simulink model "discrete_starmac"  (Simulink 6.6)
settings: Solver=FixedStepDiscrete  StartTime=0.0  StopTime=10.0  FixedStep=plant_int_period  RelTol=1e-3
values from neighbouring files (symbols this model uses):
  A = pi*R^2    (= 0.0506707479097)    [constants.m]
  b = 0.1    [constants.m]
  g = [0 0 9.8]'    [constants.m]
  J = [Jxx 0 0 ... (first row only)    [constants.m]
  K_a1s = .009    (= 0.009)    [constants.m]
  K_beta = 0.23    [constants.m]
  K_torque = 0.47    [constants.m]
  M = 1.8263    [constants.m]
  motor_noise = noise_on*(9.8/4*.05)^2    [constants.m]
  plant_int_period = t_s / tau_motor    (= 0.00131578947368)    [constants.m]
  r1 = [dx 0 -dz]'    [constants.m]
  r2 = [0 dx -dz]'    [constants.m]
  r3 = [-dx 0 -dz]'    [constants.m]
  r4 = [0 -dx -dz]'    [constants.m]
  R_90 = [0 -1 0 ... (first row only)    [constants.m]
  rho = 1.2    [constants.m]
  T_nom = M*9.8/4    (= 4.474435)    [constants.m]
  tau_motor = 10    [constants.m]
  thrust_max = 9.8 * 1    (= 9.8)    [constants.m]
  thrust_min = 0    [constants.m]
  v_min = 1e-3    (= 0.001)    [constants.m]
libraries: simulink x13, xpcmeasurementcomputinglib x5, xpclib x3, aero_sim_lib x1
settings Model: Creator=jporter  LastModifiedBy=Administrator  BufferReuse=off  ProdHWDeviceType=Generic->32-bit x86 compatible
settings DataIOCC: LimitDataPoints=off  SaveOutput=off  SignalLogging=off  SaveTime=off
settings OptimizationCC: BlockReduction=off  OptimizeBlockIOStorage=off  BufferReuse=off  ExpressionFolding=off  LocalBlockOutputs=off
settings HardwareCC: ProdIntDivRoundTo=Zero  ProdEndianess=LittleEndian  ProdHWDeviceType=Generic->32-bit x86 compatible
settings RTWCC: SystemTargetFile=xpctarget.tlc  TemplateMakefile=xpc_default_tmf  Description=xPC Target  ProcessScript=xpctarget_make_rtw_hook
settings xpcTargetCC: TargetFcnLib=ansi_tfl_table_tmw.mat  GenFloatMathFcnCalls=ANSI_C  PortableWordSizes=off  xPCisDownloadable=off

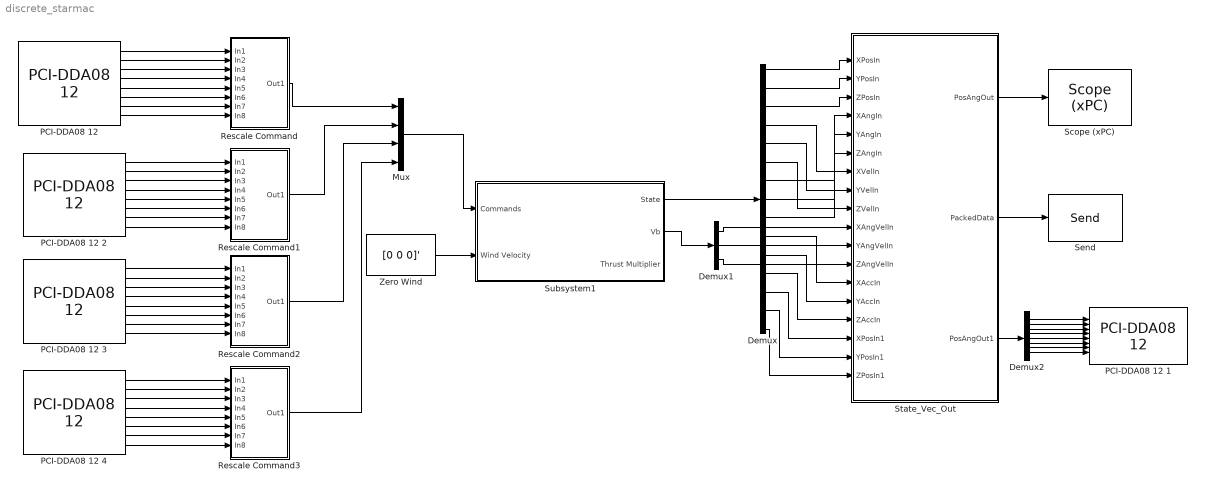
== system discrete_starmac ==
  Demux : Demux  Outputs=15
  Demux1 : Demux  Outputs=3
  Demux2 : Demux  Outputs=8
  Mux : Mux
  "PCI-DDA08 12 " : xpcmeasurementcomputinglib/Digital Input/PCI-DDA08 12   channel=[1 2 3 4 5 6 7 8]  port=A  chip=1  sampletime=plant_int_period  slot=-1
  PCI-DDA08 12 1 : xpcmeasurementcomputinglib/D//A/PCI-DDA08 12   channel=[1 2 3 4 5 6 7 8]  range=[-10 -10 -10 -10 -10 -10 -10 -10]  reset=[1]  initValue=[0]  sampletime=plant_int_period  pci_dev=-1
  PCI-DDA08 12 2 : xpcmeasurementcomputinglib/Digital Input/PCI-DDA08 12   channel=[1 2 3 4 5 6 7 8]  port=B  chip=1  sampletime=plant_int_period  slot=-1
  PCI-DDA08 12 3 : xpcmeasurementcomputinglib/Digital Input/PCI-DDA08 12   channel=[1 2 3 4 5 6 7 8]  port=A  chip=2  sampletime=plant_int_period  slot=-1
  PCI-DDA08 12 4 : xpcmeasurementcomputinglib/Digital Input/PCI-DDA08 12   channel=[1 2 3 4 5 6 7 8]  port=B  chip=2  sampletime=plant_int_period  slot=-1
  Rescale Command : Subsystem
  Rescale Command1 : Subsystem
  Rescale Command2 : Subsystem
  Rescale Command3 : Subsystem
  "Scope (xPC) " : xpclib/Misc./Scope (xPC)   SystemSampleTime=-1  scopeno=2  scopetype=Target  autostart=on  viewmode=Graphical redraw  formatstr='%15.6f'  grid=on  ylimits=[-12,12]  nosamples=250  noprepostsamples=0  interleave=1  triggermode=FreeRun  triggersignal=1  triggerlevel=0.0  triggerslope=Either  triggerscope=1  triggersample=0  filename=data.dat  mode=Lazy  writesize=512  autorestart=off
  Send : xpclib/UDP/Send  ipAddress=129.59.129.186  ipPort=9877  localPort=-1  sampletime=0.05
  State_Vec_Out : Subsystem
  Subsystem1 : Subsystem
  Zero Wind : Constant  Value=[0 0 0]'
  wires:
  Mux/1 -> Subsystem1/1(Commands)
  Zero Wind/1 -> Subsystem1/2(Wind Velocity)
  State_Vec_Out/1(PosAngOut) -> "Scope (xPC) "/1
  State_Vec_Out/2(PackedData) -> Send/1
  Subsystem1/1(State) -> Demux/1
  Demux/1 -> State_Vec_Out/1(XPosIn)
  Demux/2 -> State_Vec_Out/2(YPosIn)
  Demux/3 -> State_Vec_Out/3(ZPosIn)
  Demux/4 -> State_Vec_Out/7(XVelIn)
  Demux/5 -> State_Vec_Out/8(YVelIn)
  Demux/6 -> State_Vec_Out/9(ZVelIn)
  Demux/7 -> State_Vec_Out/4(XAngIn)
  Demux/8 -> State_Vec_Out/5(YAngIn)
  Demux/9 -> State_Vec_Out/6(ZAngIn)
  Demux/10 -> State_Vec_Out/13(XAccIn)
  Demux/11 -> State_Vec_Out/14(YAccIn)
  Demux/12 -> State_Vec_Out/15(ZAccIn)
  Demux/13 -> State_Vec_Out/16(XPosIn1)
  Demux/14 -> State_Vec_Out/17(YPosIn1)
  Demux/15 -> State_Vec_Out/18(ZPosIn1)
  Demux1/1 -> State_Vec_Out/10(XAngVelIn)
  Demux1/2 -> State_Vec_Out/11(YAngVelIn)
  Demux1/3 -> State_Vec_Out/12(ZAngVelIn)
  Subsystem1/2(Vb) -> Demux1/1
  Demux2/1 -> PCI-DDA08 12 1/1
  Demux2/2 -> PCI-DDA08 12 1/2
  Demux2/3 -> PCI-DDA08 12 1/3
  Demux2/4 -> PCI-DDA08 12 1/4
  Demux2/5 -> PCI-DDA08 12 1/5
  Demux2/6 -> PCI-DDA08 12 1/6
  Demux2/7 -> PCI-DDA08 12 1/7
  Demux2/8 -> PCI-DDA08 12 1/8
  State_Vec_Out/3(PosAngOut1) -> Demux2/1
  "PCI-DDA08 12 "/1 -> Rescale Command/1(In1)
  "PCI-DDA08 12 "/2 -> Rescale Command/2(In2)
  "PCI-DDA08 12 "/3 -> Rescale Command/3(In3)
  "PCI-DDA08 12 "/4 -> Rescale Command/4(In4)
  "PCI-DDA08 12 "/5 -> Rescale Command/5(In5)
  "PCI-DDA08 12 "/6 -> Rescale Command/6(In6)
  "PCI-DDA08 12 "/7 -> Rescale Command/7(In7)
  "PCI-DDA08 12 "/8 -> Rescale Command/8(In8)
  Rescale Command/1(Out1) -> Mux/1
  PCI-DDA08 12 2/1 -> Rescale Command1/1(In1)
  PCI-DDA08 12 2/2 -> Rescale Command1/2(In2)
  PCI-DDA08 12 2/3 -> Rescale Command1/3(In3)
  PCI-DDA08 12 2/4 -> Rescale Command1/4(In4)
  PCI-DDA08 12 2/5 -> Rescale Command1/5(In5)
  PCI-DDA08 12 2/6 -> Rescale Command1/6(In6)
  PCI-DDA08 12 2/7 -> Rescale Command1/7(In7)
  PCI-DDA08 12 2/8 -> Rescale Command1/8(In8)
  PCI-DDA08 12 3/1 -> Rescale Command2/1(In1)
  PCI-DDA08 12 3/2 -> Rescale Command2/2(In2)
  PCI-DDA08 12 3/3 -> Rescale Command2/3(In3)
  PCI-DDA08 12 3/4 -> Rescale Command2/4(In4)
  PCI-DDA08 12 3/5 -> Rescale Command2/5(In5)
  PCI-DDA08 12 3/6 -> Rescale Command2/6(In6)
  PCI-DDA08 12 3/7 -> Rescale Command2/7(In7)
  PCI-DDA08 12 3/8 -> Rescale Command2/8(In8)
  PCI-DDA08 12 4/1 -> Rescale Command3/1(In1)
  PCI-DDA08 12 4/2 -> Rescale Command3/2(In2)
  PCI-DDA08 12 4/3 -> Rescale Command3/3(In3)
  PCI-DDA08 12 4/4 -> Rescale Command3/4(In4)
  PCI-DDA08 12 4/5 -> Rescale Command3/5(In5)
  PCI-DDA08 12 4/6 -> Rescale Command3/6(In6)
  PCI-DDA08 12 4/7 -> Rescale Command3/7(In7)
  PCI-DDA08 12 4/8 -> Rescale Command3/8(In8)
  Rescale Command1/1(Out1) -> Mux/2
  Rescale Command2/1(Out1) -> Mux/3
  Rescale Command3/1(Out1) -> Mux/4

== system discrete_starmac/Rescale Command ==
  In1 : Inport  OutDataType=fixdt(1,16,0)  OutScaling=[]
  In2 : Inport  Port=2  OutDataType=fixdt(1,16,0)  OutScaling=[]
  In3 : Inport  Port=3  OutDataType=fixdt(1,16,0)  OutScaling=[]
  In4 : Inport  Port=4  OutDataType=fixdt(1,16,0)  OutScaling=[]
  In5 : Inport  Port=5  OutDataType=fixdt(1,16,0)  OutScaling=[]
  In6 : Inport  Port=6  OutDataType=fixdt(1,16,0)  OutScaling=[]
  In7 : Inport  Port=7  OutDataType=fixdt(1,16,0)  OutScaling=[]
  In8 : Inport  Port=8  OutDataType=fixdt(1,16,0)  OutScaling=[]
  Constant : Constant  Value=(2*ones(1,8)).^[7:-1:0]
  Dot Product : simulink/Math Operations/Dot Product  InputSameDT=on  OutDataType=sfix(16)  OutScaling=2^-10  DoSatur=off
  Mux1 : Mux  Inputs=8
  Rescale : Gain
  Out1 : Outport  OutDataType=fixdt(1,16,0)  OutScaling=[]
  wires:
  Mux1/1 -> Dot Product/2
  Constant/1 -> Dot Product/1
  Dot Product/1 -> Rescale/1
  In1/1 -> Mux1/1
  In2/1 -> Mux1/2
  In3/1 -> Mux1/3
  In4/1 -> Mux1/4
  In5/1 -> Mux1/5
  In6/1 -> Mux1/6
  In7/1 -> Mux1/7
  In8/1 -> Mux1/8
  Rescale/1 -> Out1/1

== system discrete_starmac/Rescale Command1 ==
  In1 : Inport  OutDataType=fixdt(1,16,0)  OutScaling=[]
  In2 : Inport  Port=2  OutDataType=fixdt(1,16,0)  OutScaling=[]
  In3 : Inport  Port=3  OutDataType=fixdt(1,16,0)  OutScaling=[]
  In4 : Inport  Port=4  OutDataType=fixdt(1,16,0)  OutScaling=[]
  In5 : Inport  Port=5  OutDataType=fixdt(1,16,0)  OutScaling=[]
  In6 : Inport  Port=6  OutDataType=fixdt(1,16,0)  OutScaling=[]
  In7 : Inport  Port=7  OutDataType=fixdt(1,16,0)  OutScaling=[]
  In8 : Inport  Port=8  OutDataType=fixdt(1,16,0)  OutScaling=[]
  Constant : Constant  Value=(2*ones(1,8)).^[7:-1:0]
  Dot Product : simulink/Math Operations/Dot Product  InputSameDT=on  OutDataType=sfix(16)  OutScaling=2^-10  DoSatur=off
  Mux1 : Mux  Inputs=8
  Rescale : Gain
  Out1 : Outport  OutDataType=fixdt(1,16,0)  OutScaling=[]
  wires:
  Mux1/1 -> Dot Product/2
  Constant/1 -> Dot Product/1
  Dot Product/1 -> Rescale/1
  In1/1 -> Mux1/1
  In2/1 -> Mux1/2
  In3/1 -> Mux1/3
  In4/1 -> Mux1/4
  In5/1 -> Mux1/5
  In6/1 -> Mux1/6
  In7/1 -> Mux1/7
  In8/1 -> Mux1/8
  Rescale/1 -> Out1/1

== system discrete_starmac/Rescale Command2 ==
  In1 : Inport  OutDataType=fixdt(1,16,0)  OutScaling=[]
  In2 : Inport  Port=2  OutDataType=fixdt(1,16,0)  OutScaling=[]
  In3 : Inport  Port=3  OutDataType=fixdt(1,16,0)  OutScaling=[]
  In4 : Inport  Port=4  OutDataType=fixdt(1,16,0)  OutScaling=[]
  In5 : Inport  Port=5  OutDataType=fixdt(1,16,0)  OutScaling=[]
  In6 : Inport  Port=6  OutDataType=fixdt(1,16,0)  OutScaling=[]
  In7 : Inport  Port=7  OutDataType=fixdt(1,16,0)  OutScaling=[]
  In8 : Inport  Port=8  OutDataType=fixdt(1,16,0)  OutScaling=[]
  Constant : Constant  Value=(2*ones(1,8)).^[7:-1:0]
  Dot Product : simulink/Math Operations/Dot Product  InputSameDT=on  OutDataType=sfix(16)  OutScaling=2^-10  DoSatur=off
  Mux1 : Mux  Inputs=8
  Rescale : Gain
  Out1 : Outport  OutDataType=fixdt(1,16,0)  OutScaling=[]
  wires:
  Mux1/1 -> Dot Product/2
  Constant/1 -> Dot Product/1
  Dot Product/1 -> Rescale/1
  In1/1 -> Mux1/1
  In2/1 -> Mux1/2
  In3/1 -> Mux1/3
  In4/1 -> Mux1/4
  In5/1 -> Mux1/5
  In6/1 -> Mux1/6
  In7/1 -> Mux1/7
  In8/1 -> Mux1/8
  Rescale/1 -> Out1/1

== system discrete_starmac/Rescale Command3 ==
  In1 : Inport  OutDataType=fixdt(1,16,0)  OutScaling=[]
  In2 : Inport  Port=2  OutDataType=fixdt(1,16,0)  OutScaling=[]
  In3 : Inport  Port=3  OutDataType=fixdt(1,16,0)  OutScaling=[]
  In4 : Inport  Port=4  OutDataType=fixdt(1,16,0)  OutScaling=[]
  In5 : Inport  Port=5  OutDataType=fixdt(1,16,0)  OutScaling=[]
  In6 : Inport  Port=6  OutDataType=fixdt(1,16,0)  OutScaling=[]
  In7 : Inport  Port=7  OutDataType=fixdt(1,16,0)  OutScaling=[]
  In8 : Inport  Port=8  OutDataType=fixdt(1,16,0)  OutScaling=[]
  Constant : Constant  Value=(2*ones(1,8)).^[7:-1:0]
  Dot Product : simulink/Math Operations/Dot Product  InputSameDT=on  OutDataType=sfix(16)  OutScaling=2^-10  DoSatur=off
  Mux1 : Mux  Inputs=8
  Rescale : Gain
  Out1 : Outport  OutDataType=fixdt(1,16,0)  OutScaling=[]
  wires:
  Mux1/1 -> Dot Product/2
  Constant/1 -> Dot Product/1
  Dot Product/1 -> Rescale/1
  In1/1 -> Mux1/1
  In2/1 -> Mux1/2
  In3/1 -> Mux1/3
  In4/1 -> Mux1/4
  In5/1 -> Mux1/5
  In6/1 -> Mux1/6
  In7/1 -> Mux1/7
  In8/1 -> Mux1/8
  Rescale/1 -> Out1/1

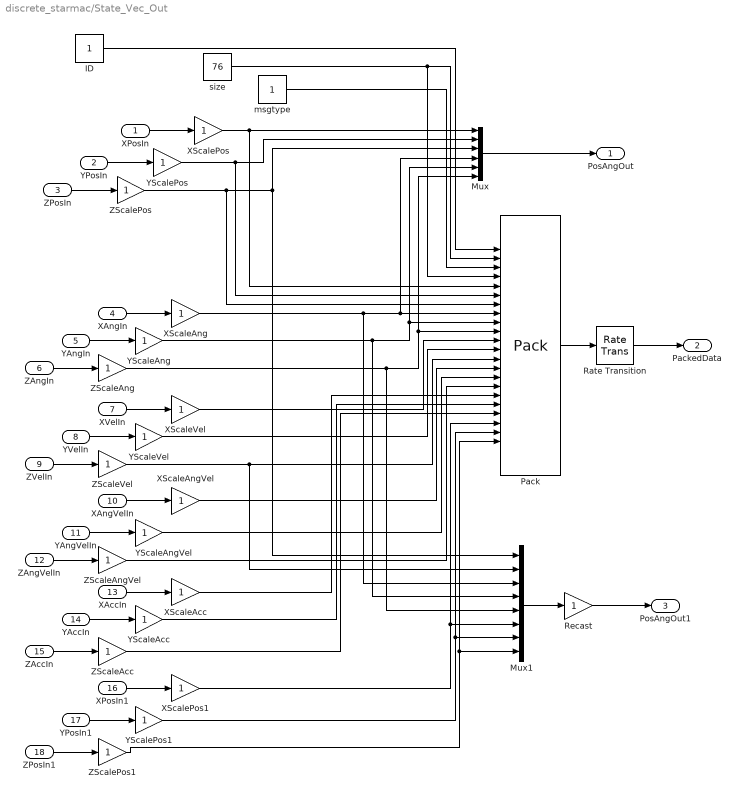
== system discrete_starmac/State_Vec_Out ==
  XPosIn : Inport
  YPosIn : Inport  Port=2
  ZPosIn : Inport  Port=3
  XAngIn : Inport  Port=4
  YAngIn : Inport  Port=5
  ZAngIn : Inport  Port=6
  XVelIn : Inport  Port=7
  YVelIn : Inport  Port=8
  ZVelIn : Inport  Port=9
  XAngVelIn : Inport  Port=10
  YAngVelIn : Inport  Port=11
  ZAngVelIn : Inport  Port=12
  XAccIn : Inport  Port=13
  YAccIn : Inport  Port=14
  ZAccIn : Inport  Port=15
  XPosIn1 : Inport  Port=16
  YPosIn1 : Inport  Port=17
  ZPosIn1 : Inport  Port=18
  ID : Constant
  Mux : Mux  Inputs=6
  Mux1 : Mux  Inputs=8
  Pack : xpclib/UDP/Pack  datatypes={'uint32','uint32','uint32','uint32','single','single','single','single','single','single','single','single','single','single','single','single','single','single','single','single','single','single'}  byteAlign=4
  Rate Transition : RateTransition
  Recast : Gain
  XScaleAcc : Gain
  XScaleAng : Gain
  XScaleAngVel : Gain
  XScalePos : Gain
  XScalePos1 : Gain
  XScaleVel : Gain
  YScaleAcc : Gain
  YScaleAng : Gain
  YScaleAngVel : Gain
  YScalePos : Gain
  YScalePos1 : Gain
  YScaleVel : Gain
  ZScaleAcc : Gain
  ZScaleAng : Gain
  ZScaleAngVel : Gain
  ZScalePos : Gain
  ZScalePos1 : Gain
  ZScaleVel : Gain
  msgtype : Constant
  size : Constant  Value=76
  PosAngOut : Outport
  PackedData : Outport  Port=2
  PosAngOut1 : Outport  Port=3
  wires:
  Pack/1 -> Rate Transition/1
  XScaleAng/1 -> Mux/4, Pack/8, Mux1/3
  YScaleAng/1 -> Mux/5, Pack/9, Mux1/4
  ZScaleAng/1 -> Mux/6, Pack/10, Mux1/5
  ID/1 -> Pack/1
  size/1 -> Pack/2, Pack/4
  msgtype/1 -> Pack/3
  XScaleVel/1 -> Pack/11
  YScaleVel/1 -> Pack/12
  ZScaleVel/1 -> Pack/13, Mux1/2
  XScaleAngVel/1 -> Pack/14
  YScaleAngVel/1 -> Pack/15
  ZScaleAngVel/1 -> Pack/16
  XScaleAcc/1 -> Pack/17
  YScaleAcc/1 -> Pack/18
  ZScaleAcc/1 -> Pack/19
  XScalePos1/1 -> Pack/20, Mux1/6
  YScalePos1/1 -> Pack/21, Mux1/7
  ZScalePos1/1 -> Pack/22, Mux1/8
  Mux/1 -> PosAngOut/1
  XPosIn/1 -> XScalePos/1
  YPosIn/1 -> YScalePos/1
  ZPosIn/1 -> ZScalePos/1
  XScalePos/1 -> Mux/1, Pack/5
  YScalePos/1 -> Mux/2, Pack/6
  ZScalePos/1 -> Pack/7, Mux/3, Mux1/1
  XAngIn/1 -> XScaleAng/1
  YAngIn/1 -> YScaleAng/1
  ZAngIn/1 -> ZScaleAng/1
  XVelIn/1 -> XScaleVel/1
  YVelIn/1 -> YScaleVel/1
  ZVelIn/1 -> ZScaleVel/1
  XAngVelIn/1 -> XScaleAngVel/1
  YAngVelIn/1 -> YScaleAngVel/1
  ZAngVelIn/1 -> ZScaleAngVel/1
  XAccIn/1 -> XScaleAcc/1
  YAccIn/1 -> YScaleAcc/1
  ZAccIn/1 -> ZScaleAcc/1
  XPosIn1/1 -> XScalePos1/1
  YPosIn1/1 -> YScalePos1/1
  ZPosIn1/1 -> ZScalePos1/1
  Rate Transition/1 -> PackedData/1
  Mux1/1 -> Recast/1
  Recast/1 -> PosAngOut1/1

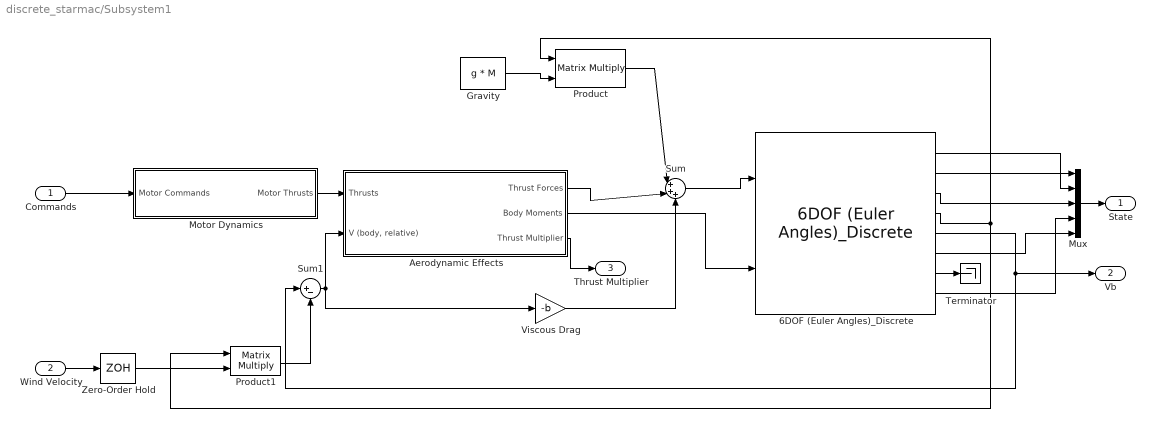
== system discrete_starmac/Subsystem1 ==
  Commands : Inport
  Wind Velocity : Inport  Port=2
  6DOF (Euler Angles)_Discrete : aero_sim_lib/6DOF (Euler Angles)_Discrete  SystemSampleTime=-1  XYZe_0=X0  Vb_0=Vb0  euler_0=T0  omega_0=W0  M=M  I=J  T_int=plant_int_period
  Aerodynamic Effects : Subsystem
  Gravity : Constant  Value=g * M
  Motor Dynamics : Subsystem
  Mux : Mux  Inputs=5
  Product : Product  Multiplication=Matrix(*)  RndMeth=Zero
  Product1 : Product  Multiplication=Matrix(*)  RndMeth=Zero
  Sum : Sum  Inputs=|+++
  Sum1 : Sum  Inputs=|+-
  Terminator : Terminator
  Viscous Drag : Gain  Gain=-b
  Zero-Order Hold : ZeroOrderHold  SampleTime=plant_int_period
  State : Outport
  Vb : Outport  Port=2
  Thrust Multiplier : Outport  Port=3
  wires:
  Motor Dynamics/1(Motor Thrusts) -> Aerodynamic Effects/1(Thrusts)
  Product/1 -> Sum/1
  Sum/1 -> 6DOF (Euler Angles)_Discrete/1
  6DOF (Euler Angles)_Discrete/4 -> Product/1, Product1/1
  Gravity/1 -> Product/2
  Sum1/1 -> Aerodynamic Effects/2("V (body, relative)"), Viscous Drag/1
  Product1/1 -> Sum1/2
  6DOF (Euler Angles)_Discrete/5 -> Sum1/1, Vb/1
  Viscous Drag/1 -> Sum/3
  6DOF (Euler Angles)_Discrete/2 -> Mux/1
  6DOF (Euler Angles)_Discrete/1 -> Mux/2
  6DOF (Euler Angles)_Discrete/3 -> Mux/3
  Aerodynamic Effects/2(Body Moments) -> 6DOF (Euler Angles)_Discrete/2
  Aerodynamic Effects/1(Thrust Forces) -> Sum/2
  Mux/1 -> State/1
  Commands/1 -> Motor Dynamics/1(Motor Commands)
  Wind Velocity/1 -> Zero-Order Hold/1
  Aerodynamic Effects/3(Thrust Multiplier) -> Thrust Multiplier/1
  6DOF (Euler Angles)_Discrete/8 -> Mux/4
  Zero-Order Hold/1 -> Product1/2
  6DOF (Euler Angles)_Discrete/7 -> Terminator/1
  6DOF (Euler Angles)_Discrete/6 -> Mux/5

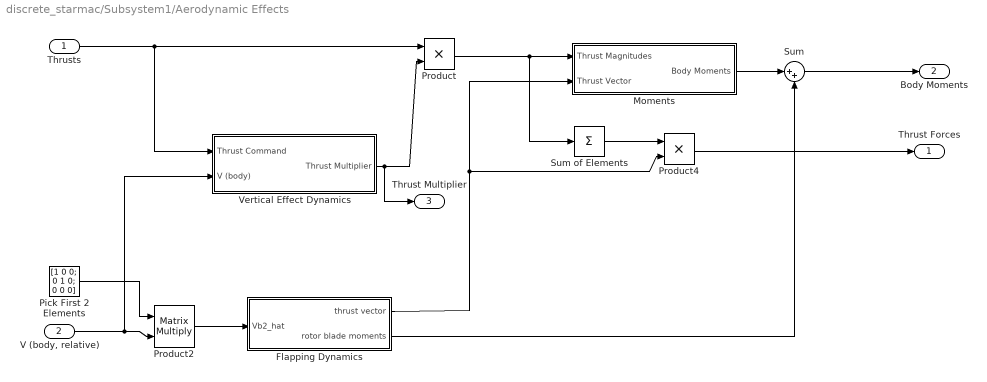
== system discrete_starmac/Subsystem1/Aerodynamic Effects ==
  Thrusts : Inport
  "V (body, relative)" : Inport  Port=2
  Flapping Dynamics : Subsystem
  Moments : Subsystem
  Pick First 2 Elements : Constant  Value=[1 0 0; 0 1 0; 0 0 0]
  Product : Product  RndMeth=Zero
  Product2 : Product  Multiplication=Matrix(*)  RndMeth=Zero
  Product4 : Product  RndMeth=Zero
  Sum : Sum  Inputs=|++
  Sum of Elements : Sum  Inputs=+  OutScaling=2^-10
  Vertical Effect Dynamics : Subsystem
  Thrust Forces : Outport
  Body Moments : Outport  Port=2
  Thrust Multiplier : Outport  Port=3
  wires:
  Thrusts/1 -> Product/1, Vertical Effect Dynamics/1(Thrust Command)
  Vertical Effect Dynamics/1(Thrust Multiplier) -> Product/2, Thrust Multiplier/1
  Product/1 -> Sum of Elements/1, Moments/1(Thrust Magnitudes)
  Pick First 2 Elements/1 -> Product2/1
  "V (body, relative)"/1 -> Product2/2, Vertical Effect Dynamics/2(V (body))
  Product2/1 -> Flapping Dynamics/1(Vb2_hat)
  Sum of Elements/1 -> Product4/1
  Product4/1 -> Thrust Forces/1
  Flapping Dynamics/1(thrust vector) -> Moments/2(Thrust Vector), Product4/2
  Moments/1(Body Moments) -> Sum/1
  Sum/1 -> Body Moments/1
  Flapping Dynamics/2(rotor blade moments) -> Sum/2

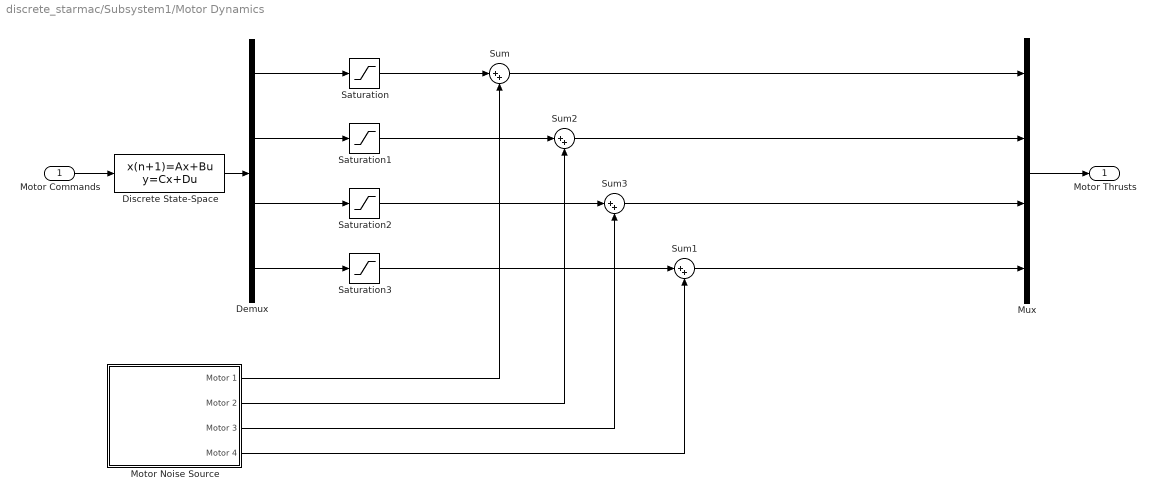
== system discrete_starmac/Subsystem1/Motor Dynamics ==
  Motor Commands : Inport
  Demux : Demux
  Discrete State-Space : DiscreteStateSpace  A=expm( -(tau_motor*plant_int_period) * eye(4) )  B=inv(expm( tau_motor * plant_int_period* eye(4))) * (expm((tau_motor*plant_int_period) * eye(4)) - eye(4))  C=eye(4)  D=zeros(4)  X0=T_nom * ones(4,1)  SampleTime=plant_int_period
  Motor Noise Source : Subsystem
  Mux : Mux
  Saturation{,1..3} (4 alike) : Saturate  UpperLimit=thrust_max  LowerLimit=thrust_min
  Sum{,1..3} (4 alike) : Sum  Inputs=|++
  Motor Thrusts : Outport
  wires:
  Demux/1 -> Saturation/1
  Demux/3 -> Saturation2/1
  Mux/1 -> Motor Thrusts/1
  Saturation/1 -> Sum/1
  Sum/1 -> Mux/1
  Saturation1/1 -> Sum2/1
  Sum2/1 -> Mux/2
  Saturation2/1 -> Sum3/1
  Sum3/1 -> Mux/3
  Saturation3/1 -> Sum1/1
  Sum1/1 -> Mux/4
  Motor Noise Source/1(Motor 1) -> Sum/2
  Motor Noise Source/2(Motor 2) -> Sum2/2
  Motor Noise Source/3(Motor 3) -> Sum3/2
  Motor Noise Source/4(Motor 4) -> Sum1/2
  Motor Commands/1 -> Discrete State-Space/1
  Discrete State-Space/1 -> Demux/1
  Demux/2 -> Saturation1/1
  Demux/4 -> Saturation3/1

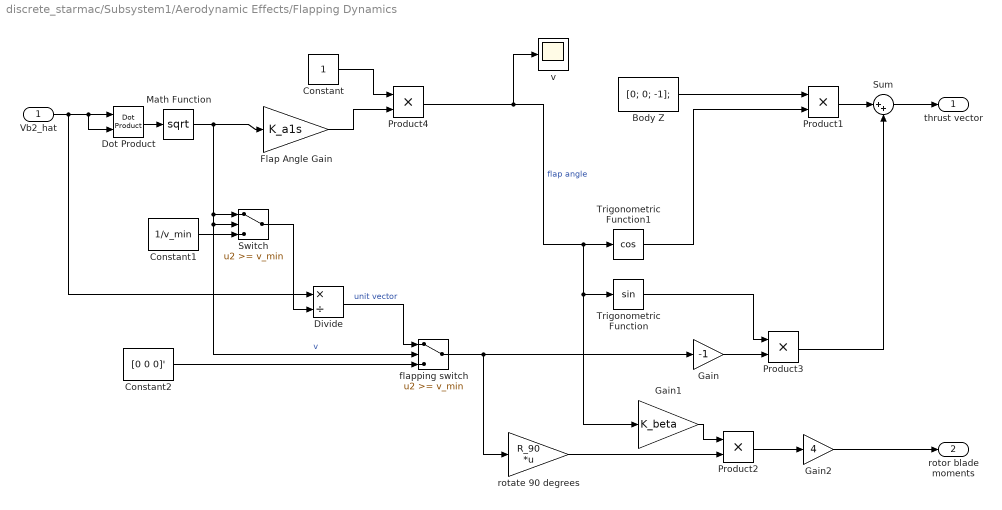
== system discrete_starmac/Subsystem1/Aerodynamic Effects/Flapping Dynamics ==
  Vb2_hat : Inport
  "Body Z " : Constant  Value=[0; 0; -1];
  Constant : Constant
  Constant1 : Constant  Value=1/v_min
  Constant2 : Constant  Value=[0 0 0]'
  Divide : Product  Inputs=*/  OutScaling=2^-10
  Dot Product : simulink/Math Operations/Dot Product  InputSameDT=on  OutDataType=sfix(16)  OutScaling=2^-10  DoSatur=off
  Flap Angle Gain : Gain  Gain=K_a1s
  Gain : Gain  Gain=-1
  Gain1 : Gain  Gain=K_beta
  Gain2 : Gain  Gain=4
  Math Function : Math  Operator=sqrt  SaturateOnIntegerOverflow=on
  Product{1..4} (4 alike) : Product  RndMeth=Zero
  Sum : Sum  Inputs=|++
  Switch : Switch  Threshold=v_min
  Trigonometric Function : Trigonometry
  Trigonometric Function1 : Trigonometry  Operator=cos
  flapping switch : Switch  Threshold=v_min
  rotate 90 degrees : Gain  Gain=R_90  Multiplication=Matrix(K*u)
  v : Scope
      settings: SaveName=ScopeData6
  thrust vector : Outport
  rotor blade moments : Outport  Port=2
  wires:
  Product4/1 -> Trigonometric Function1/1, Trigonometric Function/1, Gain1/1, v/1  "flap angle"
  Vb2_hat/1 -> Dot Product/1, Dot Product/2, Divide/1
  Dot Product/1 -> Math Function/1
  Math Function/1 -> Switch/1, Switch/2, flapping switch/2, Flap Angle Gain/1  "v"
  Trigonometric Function1/1 -> Product1/2
  Trigonometric Function/1 -> Product3/1
  Product3/1 -> Sum/2
  Gain/1 -> Product3/2
  Product1/1 -> Sum/1
  "Body Z "/1 -> Product1/1
  Sum/1 -> thrust vector/1
  Gain2/1 -> rotor blade moments/1
  Switch/1 -> Divide/2
  Constant1/1 -> Switch/3
  Divide/1 -> flapping switch/1  "unit vector"
  flapping switch/1 -> Gain/1, rotate 90 degrees/1
  Constant2/1 -> flapping switch/3
  Product2/1 -> Gain2/1
  rotate 90 degrees/1 -> Product2/2
  Gain1/1 -> Product2/1
  Flap Angle Gain/1 -> Product4/2
  Constant/1 -> Product4/1

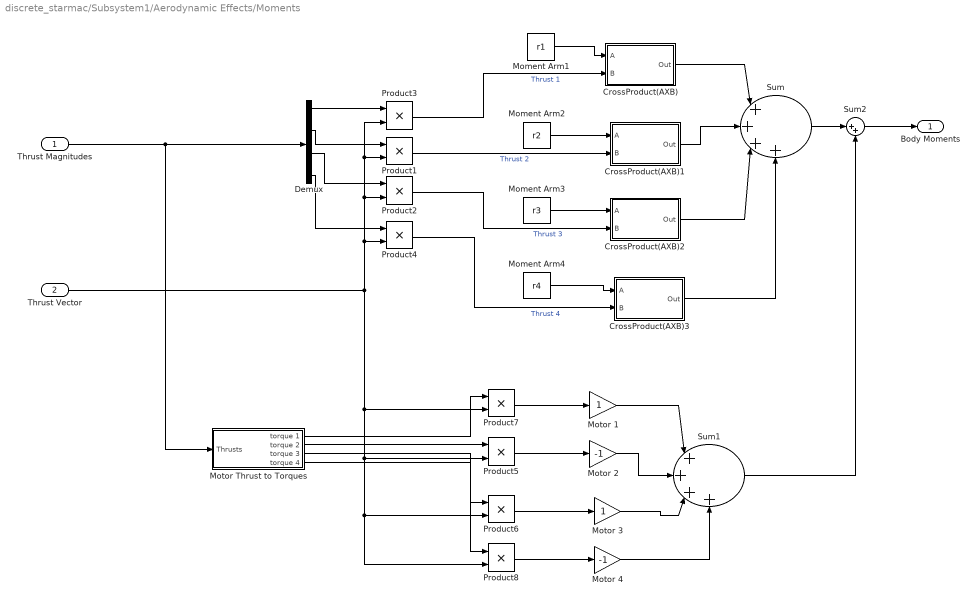
== system discrete_starmac/Subsystem1/Aerodynamic Effects/Moments ==
  Thrust Magnitudes : Inport
  Thrust Vector : Inport  Port=2
  CrossProduct(AXB) : Subsystem
  CrossProduct(AXB)1 : Subsystem
  CrossProduct(AXB)2 : Subsystem
  CrossProduct(AXB)3 : Subsystem
  Demux : Demux
  Moment Arm1 : Constant  Value=r1
  Moment Arm2 : Constant  Value=r2
  Moment Arm3 : Constant  Value=r3
  Moment Arm4 : Constant  Value=r4
  Motor 1 : Gain
  Motor 2 : Gain  Gain=-1
  Motor 3 : Gain
  Motor 4 : Gain  Gain=-1
  Motor Thrust to Torques : Subsystem
  Product{1..8} (8 alike) : Product  RndMeth=Zero
  Sum : Sum  Inputs=|++++
  Sum1 : Sum  Inputs=|++++
  Sum2 : Sum  Inputs=|++
  Body Moments : Outport
  wires:
  Thrust Magnitudes/1 -> Demux/1, Motor Thrust to Torques/1(Thrusts)
  Demux/1 -> Product3/1
  Demux/2 -> Product1/1
  Demux/3 -> Product2/1
  Demux/4 -> Product4/1
  Thrust Vector/1 -> Product3/2, Product1/2, Product2/2, Product4/2, Product7/2, Product5/2, Product6/2, Product8/2
  Moment Arm1/1 -> CrossProduct(AXB)/1(A)
  Product3/1 -> CrossProduct(AXB)/2(B)  "Thrust 1"
  Moment Arm2/1 -> CrossProduct(AXB)1/1(A)
  Product1/1 -> CrossProduct(AXB)1/2(B)  "Thrust 2"
  Moment Arm3/1 -> CrossProduct(AXB)2/1(A)
  Product2/1 -> CrossProduct(AXB)2/2(B)  "Thrust 3"
  Moment Arm4/1 -> CrossProduct(AXB)3/1(A)
  Product4/1 -> CrossProduct(AXB)3/2(B)  "Thrust 4"
  CrossProduct(AXB)/1(Out) -> Sum/1
  CrossProduct(AXB)2/1(Out) -> Sum/3
  CrossProduct(AXB)3/1(Out) -> Sum/4
  Motor 1/1 -> Sum1/1
  Motor 2/1 -> Sum1/2
  Motor 3/1 -> Sum1/3
  Motor 4/1 -> Sum1/4
  Sum/1 -> Sum2/1
  Sum1/1 -> Sum2/2
  Sum2/1 -> Body Moments/1
  Product7/1 -> Motor 1/1
  Product5/1 -> Motor 2/1
  Product6/1 -> Motor 3/1
  Product8/1 -> Motor 4/1
  Motor Thrust to Torques/1(torque 1) -> Product7/1
  Motor Thrust to Torques/2(torque 2) -> Product5/1
  Motor Thrust to Torques/3(torque 3) -> Product6/1
  Motor Thrust to Torques/4(torque 4) -> Product8/1
  CrossProduct(AXB)1/1(Out) -> Sum/2

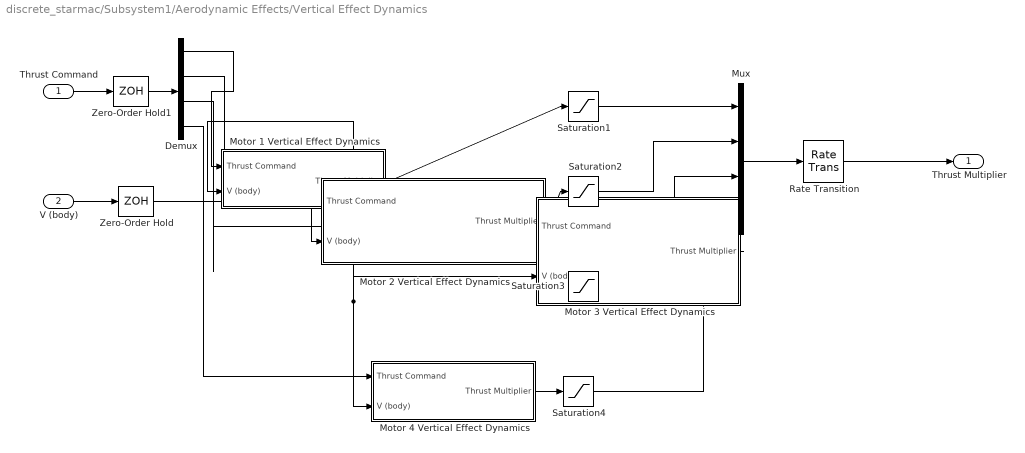
== system discrete_starmac/Subsystem1/Aerodynamic Effects/Vertical Effect Dynamics ==
  Thrust Command : Inport
  V (body) : Inport  Port=2
  Demux : Demux
  Motor 1 Vertical Effect Dynamics : Subsystem
  Motor 2 Vertical Effect Dynamics : Subsystem
  Motor 3 Vertical Effect Dynamics : Subsystem
  Motor 4 Vertical Effect Dynamics : Subsystem
  Mux : Mux
  Rate Transition : RateTransition
  Saturation{1..4} (4 alike) : Saturate  UpperLimit=2  LowerLimit=0.5
  Zero-Order Hold : ZeroOrderHold  SampleTime=plant_int_period*10
  Zero-Order Hold1 : ZeroOrderHold  SampleTime=plant_int_period*10
  Thrust Multiplier : Outport
  wires:
  Thrust Command/1 -> Zero-Order Hold1/1
  Mux/1 -> Rate Transition/1
  Demux/1 -> Motor 1 Vertical Effect Dynamics/1(Thrust Command)
  Demux/2 -> Motor 2 Vertical Effect Dynamics/1(Thrust Command)
  Demux/3 -> Motor 3 Vertical Effect Dynamics/1(Thrust Command)
  Demux/4 -> Motor 4 Vertical Effect Dynamics/1(Thrust Command)
  Motor 1 Vertical Effect Dynamics/1(Thrust Multiplier) -> Saturation1/1
  Motor 2 Vertical Effect Dynamics/1(Thrust Multiplier) -> Saturation2/1
  Motor 3 Vertical Effect Dynamics/1(Thrust Multiplier) -> Saturation3/1
  Motor 4 Vertical Effect Dynamics/1(Thrust Multiplier) -> Saturation4/1
  Saturation1/1 -> Mux/1
  Saturation2/1 -> Mux/2
  Saturation3/1 -> Mux/3
  Saturation4/1 -> Mux/4
  V (body)/1 -> Zero-Order Hold/1
  Zero-Order Hold/1 -> Motor 1 Vertical Effect Dynamics/2(V (body)), Motor 2 Vertical Effect Dynamics/2(V (body)), Motor 3 Vertical Effect Dynamics/2(V (body)), Motor 4 Vertical Effect Dynamics/2(V (body))
  Zero-Order Hold1/1 -> Demux/1
  Rate Transition/1 -> Thrust Multiplier/1

== system discrete_starmac/Subsystem1/Motor Dynamics/Motor Noise Source ==
  Motor Noise : RandomNumber  Variance=motor_noise  SampleTime=plant_int_period
  Motor Noise1 : RandomNumber  Variance=motor_noise  Seed=1  SampleTime=plant_int_period
  Motor Noise2 : RandomNumber  Variance=motor_noise  Seed=2  SampleTime=plant_int_period
  Motor Noise3 : RandomNumber  Variance=motor_noise  Seed=3  SampleTime=plant_int_period
  Motor 1 : Outport
  Motor 2 : Outport  Port=2
  Motor 3 : Outport  Port=3
  Motor 4 : Outport  Port=4
  wires:
  Motor Noise/1 -> Motor 1/1
  Motor Noise1/1 -> Motor 2/1
  Motor Noise2/1 -> Motor 3/1
  Motor Noise3/1 -> Motor 4/1

== system discrete_starmac/Subsystem1/Aerodynamic Effects/Moments/CrossProduct(AXB) ==
  A : Inport
  B : Inport  Port=2
  Fcn : Fcn  Expr=u[2]*u[6]-u[3]*u[5]
  Fcn1 : Fcn  Expr=u[3]*u[4]-u[1]*u[6]
  Fcn2 : Fcn  Expr=u[1]*u[5]-u[2]*u[4]
  Mux : Mux  Inputs=2
  Mux1 : Mux  Inputs=3
  Out : Outport
  wires:
  A/1 -> Mux/1
  B/1 -> Mux/2
  Mux/1 -> Fcn/1, Fcn1/1, Fcn2/1
  Fcn/1 -> Mux1/1
  Fcn1/1 -> Mux1/2
  Fcn2/1 -> Mux1/3
  Mux1/1 -> Out/1

== system discrete_starmac/Subsystem1/Aerodynamic Effects/Moments/CrossProduct(AXB)1 ==
  A : Inport
  B : Inport  Port=2
  Fcn : Fcn  Expr=u[2]*u[6]-u[3]*u[5]
  Fcn1 : Fcn  Expr=u[3]*u[4]-u[1]*u[6]
  Fcn2 : Fcn  Expr=u[1]*u[5]-u[2]*u[4]
  Mux : Mux  Inputs=2
  Mux1 : Mux  Inputs=3
  Out : Outport
  wires:
  Mux1/1 -> Out/1
  Fcn2/1 -> Mux1/3
  Fcn1/1 -> Mux1/2
  Fcn/1 -> Mux1/1
  Mux/1 -> Fcn2/1, Fcn1/1, Fcn/1
  B/1 -> Mux/2
  A/1 -> Mux/1

== system discrete_starmac/Subsystem1/Aerodynamic Effects/Moments/CrossProduct(AXB)2 ==
  A : Inport
  B : Inport  Port=2
  Fcn : Fcn  Expr=u[2]*u[6]-u[3]*u[5]
  Fcn1 : Fcn  Expr=u[3]*u[4]-u[1]*u[6]
  Fcn2 : Fcn  Expr=u[1]*u[5]-u[2]*u[4]
  Mux : Mux  Inputs=2
  Mux1 : Mux  Inputs=3
  Out : Outport
  wires:
  A/1 -> Mux/1
  B/1 -> Mux/2
  Mux/1 -> Fcn/1, Fcn1/1, Fcn2/1
  Fcn/1 -> Mux1/1
  Fcn1/1 -> Mux1/2
  Fcn2/1 -> Mux1/3
  Mux1/1 -> Out/1

== system discrete_starmac/Subsystem1/Aerodynamic Effects/Moments/CrossProduct(AXB)3 ==
  A : Inport
  B : Inport  Port=2
  Fcn : Fcn  Expr=u[2]*u[6]-u[3]*u[5]
  Fcn1 : Fcn  Expr=u[3]*u[4]-u[1]*u[6]
  Fcn2 : Fcn  Expr=u[1]*u[5]-u[2]*u[4]
  Mux : Mux  Inputs=2
  Mux1 : Mux  Inputs=3
  Out : Outport
  wires:
  Mux1/1 -> Out/1
  Fcn2/1 -> Mux1/3
  Fcn1/1 -> Mux1/2
  Fcn/1 -> Mux1/1
  Mux/1 -> Fcn2/1, Fcn1/1, Fcn/1
  B/1 -> Mux/2
  A/1 -> Mux/1

== system discrete_starmac/Subsystem1/Aerodynamic Effects/Moments/Motor Thrust to Torques ==
  Thrusts : Inport
  Demux : Demux
  Gain1 : Gain  Gain=K_torque
  torque 1 : Outport
  torque 2 : Outport  Port=2
  torque 3 : Outport  Port=3
  torque 4 : Outport  Port=4
  wires:
  Thrusts/1 -> Gain1/1
  Gain1/1 -> Demux/1
  Demux/1 -> torque 1/1
  Demux/2 -> torque 2/1
  Demux/3 -> torque 3/1
  Demux/4 -> torque 4/1

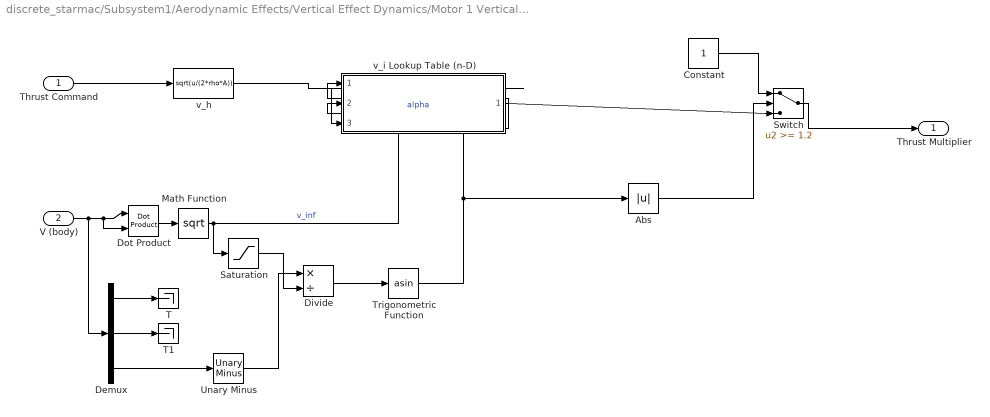
== system discrete_starmac/Subsystem1/Aerodynamic Effects/Vertical Effect Dynamics/Motor 1 Vertical Effect Dynamics ==
  Thrust Command : Inport
  V (body) : Inport  Port=2
  Abs : Abs
  Constant : Constant
  Demux : Demux  Outputs=3
  Divide : Product  Inputs=*/  OutScaling=2^-10
  Dot Product : simulink/Math Operations/Dot Product  InputSameDT=on  OutDataType=sfix(16)  OutScaling=2^-10  DoSatur=off
  Math Function : Math  Operator=sqrt  SaturateOnIntegerOverflow=on
  Saturation : Saturate  UpperLimit=500000  LowerLimit=0.0000000001
  Switch : Switch  Threshold=1.2
  T : Terminator
  T1 : Terminator
  Trigonometric Function : Trigonometry  Operator=asin
  Unary Minus : simulink/Math Operations/Unary Minus  DoSatur=off
  "v_h " : Fcn  Expr=sqrt(u/(2*rho*A))
  v_i Lookup Table (n-D) : Subsystem
  Thrust Multiplier : Outport
  wires:
  Thrust Command/1 -> "v_h "/1
  V (body)/1 -> Dot Product/1, Dot Product/2, Demux/1
  "v_h "/1 -> v_i Lookup Table (n-D)/3
  Dot Product/1 -> Math Function/1
  Math Function/1 -> Saturation/1, v_i Lookup Table (n-D)/2  "v_inf"
  Demux/1 -> T/1
  Demux/2 -> T1/1
  Divide/1 -> Trigonometric Function/1
  Trigonometric Function/1 -> Abs/1, v_i Lookup Table (n-D)/1  "alpha"
  Switch/1 -> Thrust Multiplier/1
  v_i Lookup Table (n-D)/1 -> Switch/3
  Constant/1 -> Switch/1
  Abs/1 -> Switch/2
  Unary Minus/1 -> Divide/1
  Demux/3 -> Unary Minus/1
  Saturation/1 -> Divide/2

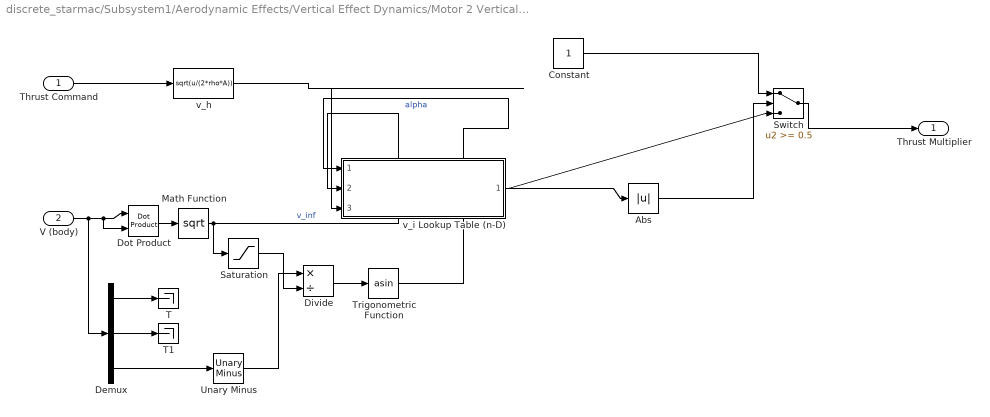
== system discrete_starmac/Subsystem1/Aerodynamic Effects/Vertical Effect Dynamics/Motor 2 Vertical Effect Dynamics ==
  Thrust Command : Inport
  V (body) : Inport  Port=2
  Abs : Abs
  Constant : Constant
  Demux : Demux  Outputs=3
  Divide : Product  Inputs=*/  OutScaling=2^-10
  Dot Product : simulink/Math Operations/Dot Product  InputSameDT=on  OutDataType=sfix(16)  OutScaling=2^-10  DoSatur=off
  Math Function : Math  Operator=sqrt  SaturateOnIntegerOverflow=on
  Saturation : Saturate  UpperLimit=500000  LowerLimit=0.00001
  Switch : Switch  Threshold=0.5
  T : Terminator
  T1 : Terminator
  Trigonometric Function : Trigonometry  Operator=asin
  Unary Minus : simulink/Math Operations/Unary Minus  DoSatur=off
  "v_h " : Fcn  Expr=sqrt(u/(2*rho*A))
  v_i Lookup Table (n-D) : Subsystem
  Thrust Multiplier : Outport
  wires:
  Thrust Command/1 -> "v_h "/1
  V (body)/1 -> Dot Product/1, Dot Product/2, Demux/1
  "v_h "/1 -> v_i Lookup Table (n-D)/3
  Dot Product/1 -> Math Function/1
  Math Function/1 -> Saturation/1, v_i Lookup Table (n-D)/2  "v_inf"
  Demux/1 -> T/1
  Demux/2 -> T1/1
  Divide/1 -> Trigonometric Function/1
  Trigonometric Function/1 -> Abs/1, v_i Lookup Table (n-D)/1  "alpha"
  Switch/1 -> Thrust Multiplier/1
  v_i Lookup Table (n-D)/1 -> Switch/3
  Constant/1 -> Switch/1
  Abs/1 -> Switch/2
  Unary Minus/1 -> Divide/1
  Demux/3 -> Unary Minus/1
  Saturation/1 -> Divide/2

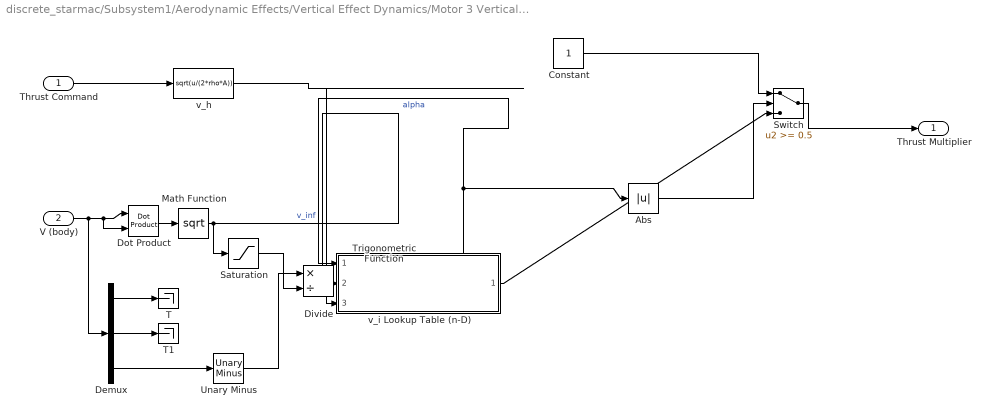
== system discrete_starmac/Subsystem1/Aerodynamic Effects/Vertical Effect Dynamics/Motor 3 Vertical Effect Dynamics ==
  Thrust Command : Inport
  V (body) : Inport  Port=2
  Abs : Abs
  Constant : Constant
  Demux : Demux  Outputs=3
  Divide : Product  Inputs=*/  OutScaling=2^-10
  Dot Product : simulink/Math Operations/Dot Product  InputSameDT=on  OutDataType=sfix(16)  OutScaling=2^-10  DoSatur=off
  Math Function : Math  Operator=sqrt  SaturateOnIntegerOverflow=on
  Saturation : Saturate  UpperLimit=500000  LowerLimit=0.00001
  Switch : Switch  Threshold=0.5
  T : Terminator
  T1 : Terminator
  Trigonometric Function : Trigonometry  Operator=asin
  Unary Minus : simulink/Math Operations/Unary Minus  DoSatur=off
  "v_h " : Fcn  Expr=sqrt(u/(2*rho*A))
  v_i Lookup Table (n-D) : Subsystem
  Thrust Multiplier : Outport
  wires:
  Thrust Command/1 -> "v_h "/1
  V (body)/1 -> Dot Product/1, Dot Product/2, Demux/1
  "v_h "/1 -> v_i Lookup Table (n-D)/3
  Dot Product/1 -> Math Function/1
  Math Function/1 -> Saturation/1, v_i Lookup Table (n-D)/2  "v_inf"
  Demux/1 -> T/1
  Demux/2 -> T1/1
  Divide/1 -> Trigonometric Function/1
  Trigonometric Function/1 -> Abs/1, v_i Lookup Table (n-D)/1  "alpha"
  Switch/1 -> Thrust Multiplier/1
  v_i Lookup Table (n-D)/1 -> Switch/3
  Constant/1 -> Switch/1
  Abs/1 -> Switch/2
  Unary Minus/1 -> Divide/1
  Demux/3 -> Unary Minus/1
  Saturation/1 -> Divide/2

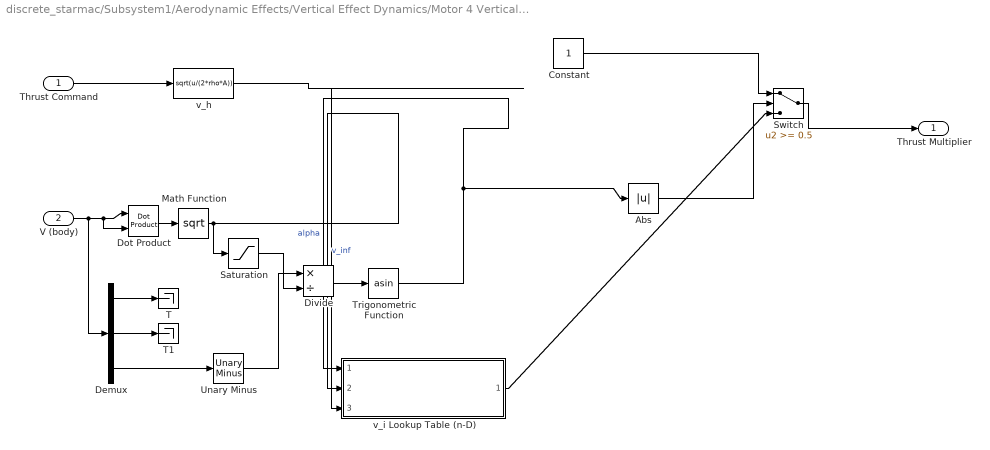
== system discrete_starmac/Subsystem1/Aerodynamic Effects/Vertical Effect Dynamics/Motor 4 Vertical Effect Dynamics ==
  Thrust Command : Inport
  V (body) : Inport  Port=2
  Abs : Abs
  Constant : Constant
  Demux : Demux  Outputs=3
  Divide : Product  Inputs=*/  OutScaling=2^-10
  Dot Product : simulink/Math Operations/Dot Product  InputSameDT=on  OutDataType=sfix(16)  OutScaling=2^-10  DoSatur=off
  Math Function : Math  Operator=sqrt  SaturateOnIntegerOverflow=on
  Saturation : Saturate  UpperLimit=500000  LowerLimit=0.00001
  Switch : Switch  Threshold=0.5
  T : Terminator
  T1 : Terminator
  Trigonometric Function : Trigonometry  Operator=asin
  Unary Minus : simulink/Math Operations/Unary Minus  DoSatur=off
  "v_h " : Fcn  Expr=sqrt(u/(2*rho*A))
  v_i Lookup Table (n-D) : Subsystem
  Thrust Multiplier : Outport
  wires:
  Thrust Command/1 -> "v_h "/1
  V (body)/1 -> Dot Product/1, Dot Product/2, Demux/1
  "v_h "/1 -> v_i Lookup Table (n-D)/3
  Dot Product/1 -> Math Function/1
  Math Function/1 -> Saturation/1, v_i Lookup Table (n-D)/2  "v_inf"
  Demux/1 -> T/1
  Demux/2 -> T1/1
  Divide/1 -> Trigonometric Function/1
  Trigonometric Function/1 -> Abs/1, v_i Lookup Table (n-D)/1  "alpha"
  Switch/1 -> Thrust Multiplier/1
  v_i Lookup Table (n-D)/1 -> Switch/3
  Constant/1 -> Switch/1
  Abs/1 -> Switch/2
  Unary Minus/1 -> Divide/1
  Demux/3 -> Unary Minus/1
  Saturation/1 -> Divide/2

== system discrete_starmac/Subsystem1/Aerodynamic Effects/Vertical Effect Dynamics/Motor 1 Vertical Effect Dynamics/v_i Lookup Table (n-D) ==

== system discrete_starmac/Subsystem1/Aerodynamic Effects/Vertical Effect Dynamics/Motor 2 Vertical Effect Dynamics/v_i Lookup Table (n-D) ==

== system discrete_starmac/Subsystem1/Aerodynamic Effects/Vertical Effect Dynamics/Motor 3 Vertical Effect Dynamics/v_i Lookup Table (n-D) ==

== system discrete_starmac/Subsystem1/Aerodynamic Effects/Vertical Effect Dynamics/Motor 4 Vertical Effect Dynamics/v_i Lookup Table (n-D) ==
